simulink model "inicio_do_sistema"  (R2023b)
settings: Solver=FixedStepAuto  StartTime=0.0  StopTime=5.0  FixedStep=Te1  RelTol=1e-3
values from neighbouring files (symbols this model uses):
  Am = [-1/tau 0; 1 0]    [InitCommande_Aero.m]
  B1m = [Kv/tau ; 0]    [InitCommande_Aero.m]
  Cm = [1 0]    [InitCommande_Aero.m]
  Kw = Ka(1)    [InitCommande_Aero.m]    (also in matlab_variables_2_2.mat = 0.240350108962)
  Kz = Ka(2)    [InitCommande_Aero.m]    (also in matlab_variables_2_2.mat = 4.57892915652)
settings Model: Creator=rick  LastModifiedBy=rick
settings DataIOCC: SaveFormat=Array  ReturnWorkspaceOutputs=off

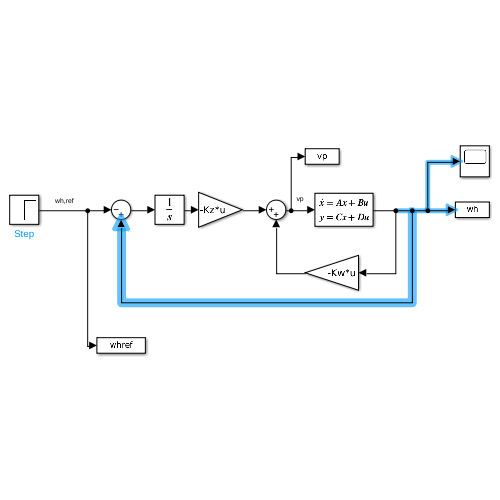
[thumbnail: Simulink's stored preview of the top-level diagram]
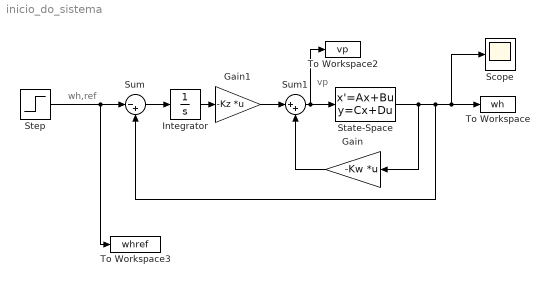
== system inicio_do_sistema ==
  note: vp
  note: wh,ref
  Gain : Gain  Gain=-Kw  Multiplication=Matrix(K*u)
  Gain1 : Gain  Gain=-Kz  Multiplication=Matrix(K*u)
  Integrator : Integrator
  Scope : Scope
  State-Space : StateSpace  A=Am  B=B1m  C=Cm  D=0  InitialCondition=0
  Step : Step  After=150  SampleTime=0
  Sum : Sum  Inputs=|-+
  Sum1 : Sum  Inputs=|++
  To Workspace : ToWorkspace  VariableName=wh  SampleTime=-1
  To Workspace2 : ToWorkspace  VariableName=vp  SampleTime=-1
      settings: Save2DSignal=2-D array (concatenate along first dimension)
  To Workspace3 : ToWorkspace  VariableName=whref  SampleTime=-1
  wires:
  Step/1 -> Sum/1, To Workspace3/1
  Gain/1 -> Sum1/2
  State-Space/1 -> Sum/2, To Workspace/1, Scope/1, Gain/1
  Sum/1 -> Integrator/1
  Sum1/1 -> To Workspace2/1, State-Space/1
  Integrator/1 -> Gain1/1
  Gain1/1 -> Sum1/1
